simulink model "exampleModel_bus_axi"  (R2017b)
settings: Solver=VariableStepAuto  StartTime=0.0  StopTime=3e-5  RelTol=1e-3
PreLoadFcn:
  | setup
values from neighbouring files (symbols this model uses):
  axiClk = 156.25e6    (= 156250000)    [setup.m]    (also in setup_exampleModel_bus_axi_simulink.m; setup_exampleModel_bus_axi_simulink_lcls2.m; setup_lcls2_pcav.m; sysgen_signal.m)
  cav1p1_addr = 204    [setup_exampleModel_bus_axi_simulink.m]    (also in setup_exampleModel_bus_axi_simulink_lcls2.m; setup_lcls2_pcav.m; sysgen_signal.m)
  cav1p2_addr = cav1p1_addr * 2    (= 408)    [setup_exampleModel_bus_axi_simulink.m]    (also in setup_exampleModel_bus_axi_simulink_lcls2.m; setup_lcls2_pcav.m; sysgen_signal.m)
  cav2p1_addr = cav1p1_addr * 3    (= 612)    [setup_exampleModel_bus_axi_simulink.m]    (also in setup_exampleModel_bus_axi_simulink_lcls2.m; setup_lcls2_pcav.m; sysgen_signal.m)
  cav2p2_addr = cav1p1_addr * 4    (= 816)    [setup_exampleModel_bus_axi_simulink.m]    (also in setup_exampleModel_bus_axi_simulink_lcls2.m; setup_lcls2_pcav.m; sysgen_signal.m)
  Fadc = Fs/interleavedChannels    (= 29750000)    [setup.m]    (also in setup_exampleModel_bus_axi_simulink.m = 357000000; setup_exampleModel_bus_axi_simulink_lcls2.m = 351000000; setup_lcls2_pcav.m = 357000000; sysgen_signal.m = 357000000)
  Fproc = 204e6    (= 204000000)    [setup_exampleModel_bus_axi_simulink.m]    (also in setup_exampleModel_bus_axi_simulink_lcls2.m = 200571400; setup_lcls2_pcav.m; sysgen_signal.m)
  Fsig = Fproc/12    (= 17000000)    [setup_exampleModel_bus_axi_simulink.m]    (also in setup_exampleModel_bus_axi_simulink_lcls2.m = 16714283.3333; setup_lcls2_pcav.m)
  Tadc = 1/fadc    (= 2.80112044818e-09)    [cavity_signal.m]    (also in setup_exampleModel_bus_axi_simulink.m; setup_exampleModel_bus_axi_simulink_lcls2.m = 2.849002849e-09; setup_lcls2_pcav.m; setup_pcav_simulink.m)
undefined symbols (not defined in the file or in its folder): AXI4, Lite
libraries: xbsIndex_r4 x2037, llrf_lib x10, simulink x1
(part 11 of 12)

== system exampleModel_bus_axi/example/dsp/Cav1/c1p2_freq_err_module1/freq_err1/delta_phi ==
  note: calculating delta phi
  phase : Inport
  window : Inport  Port=2
  reset : Inport  Port=3
  AddSub3 : xbsIndex_r4/AddSub  mode=Subtraction  use_carryin=off  use_carryout=off  en=on  latency=1  precision=Full  arith_type="Signed  (2's comp)"  n_bits=32  bin_pt=30  quantization=Truncate  overflow=Saturate  use_behavioral_HDL=off  hw_selection=Fabric  pipelined=off  dbl_ovrd=off  block_type=addsub
  Constant : xbsIndex_r4/Constant  const=0  gui_display_data_type=Fixed-point  arith_type=Signed (2's comp)  n_bits=1  bin_pt=0  preci_type=Single  exp_width=8  frac_width=24  explicit_period=off  period=1  equ=P=C  opselect=C  inp2=PCIN>>17  opr=+  inp1=P  carry=CIN  dbl_ovrd=off  block_type=constant
  Constant1 : xbsIndex_r4/Constant  const=0  gui_display_data_type=Fixed-point  arith_type=Signed (2's comp)  n_bits=1  bin_pt=0  preci_type=Single  exp_width=8  frac_width=24  explicit_period=off  period=1  equ=P=C  opselect=C  inp2=PCIN>>17  opr=+  inp1=P  carry=CIN  dbl_ovrd=off  block_type=constant
  Convert1 : xbsIndex_r4/Convert  gui_display_data_type=Boolean  arith_type=Boolean  n_bits=16  bin_pt=14  float_type=Single  exp_bits=8  fraction_bits=24  quantization=Truncate  overflow=Wrap  en=off  latency=1  pipeline=off  dbl_ovrd=off  block_type=convert
  Delay : xbsIndex_r4/Delay  rst=off  infoeditControl=Selection of Reset will increase slice count due to use of real FFs and instead of SRLs  en=off  latency=5  reg_retiming=off  dbl_ovrd=off  block_type=delay
  Delay2 : xbsIndex_r4/Delay  rst=off  infoeditControl=Selection of Reset will increase slice count due to use of real FFs and instead of SRLs  en=off  latency=2  reg_retiming=off  dbl_ovrd=off  block_type=delay
  Display : Display
  Display1 : Display
  Display2 : Display
  Gateway Out27 : xbsIndex_r4/Gateway Out  inherit_from_input=off  hdl_port=on  rows=1  columns=1  UseAsDAC=off  DACChannel='1'  interface=None  automatic_assignment=on  address_offset=hex2dec('00')  intf_name=''  intf_description=''  timing_constraint=None  locs_specified=off  LOCs={}  io_standard={}  block_type=gatewayout
  Gateway Out28 : xbsIndex_r4/Gateway Out  inherit_from_input=off  hdl_port=on  rows=1  columns=1  UseAsDAC=off  DACChannel='1'  interface=None  automatic_assignment=on  address_offset=hex2dec('00')  intf_name=''  intf_description=''  timing_constraint=None  locs_specified=off  LOCs={}  io_standard={}  block_type=gatewayout
  Gateway Out29 : xbsIndex_r4/Gateway Out  inherit_from_input=off  hdl_port=on  rows=1  columns=1  UseAsDAC=off  DACChannel='1'  interface=None  automatic_assignment=on  address_offset=hex2dec('00')  intf_name=''  intf_description=''  timing_constraint=None  locs_specified=off  LOCs={}  io_standard={}  block_type=gatewayout
  Inverter : xbsIndex_r4/Inverter  en=off  latency=1  dbl_ovrd=off  block_type=inv
  Logical : xbsIndex_r4/Logical  logical_function=AND  inputs=2  en=off  latency=7  precision=User Defined  arith_type=Boolean  n_bits=1  bin_pt=0  align_bp=on  dbl_ovrd=off  block_type=logical
  Relational : xbsIndex_r4/Relational  mode=a!=b  op_type=Bool  en=off  latency=1  dbl_ovrd=off  block_type=relational
  Relational1 : xbsIndex_r4/Relational  mode=a!=b  op_type=Bool  en=off  latency=1  dbl_ovrd=off  block_type=relational
  low_bit : Scope  NumInputPorts=4
  phase_latching : Subsystem
  posedge_pulse : Subsystem
  d_phi : Outport
  val_latched : Outport  Port=2
  wires:
  Delay/1 -> val_latched/1
  posedge_pulse/1(Out1) -> Delay/1
  reset/1 -> phase_latching/3(reset)
  Inverter/1 -> Delay2/1
  Delay2/1 -> AddSub3/3
  Gateway Out29/1 -> low_bit/1, Display/1
  phase/1 -> phase_latching/1(phase)
  AddSub3/1 -> Gateway Out27/1, d_phi/1
  Gateway Out28/1 -> low_bit/2, Display1/1
  Gateway Out27/1 -> low_bit/3, Display2/1
  Convert1/1 -> Inverter/1
  window/1 -> Convert1/1, phase_latching/2(window)
  phase_latching/1(Stop_value) -> AddSub3/1, Relational/1, Gateway Out29/1
  Constant/1 -> Relational/2
  Constant1/1 -> Relational1/2
  phase_latching/2(Start_value) -> Relational1/1, Gateway Out28/1, AddSub3/2
  Relational/1 -> Logical/1
  Relational1/1 -> Logical/2
  Logical/1 -> posedge_pulse/1(In1)

== system exampleModel_bus_axi/example/dsp/Cav1/c1p2_freq_err_module1/freq_err1/delta_t ==
  note: (2*pi)/(17E6)
  window : Inport
  reset : Inport  Port=2
  Constant1 : xbsIndex_r4/Constant  const=2*pi*(1/(Fsig))  gui_display_data_type=Fixed-point  arith_type=Unsigned  n_bits=42  bin_pt=42  preci_type=Single  exp_width=8  frac_width=24  explicit_period=off  period=1  equ=P=C  opselect=C  inp2=PCIN>>17  opr=+  inp1=P  carry=CIN  dbl_ovrd=off  block_type=constant
  Convert1 : xbsIndex_r4/Convert  gui_display_data_type=Boolean  arith_type=Boolean  n_bits=16  bin_pt=14  float_type=Single  exp_bits=8  fraction_bits=24  quantization=Truncate  overflow=Wrap  en=off  latency=1  pipeline=off  dbl_ovrd=off  block_type=convert
  Counter2 : xbsIndex_r4/Counter  cnt_type=Free Running  cnt_to=Inf  operation=Up  start_count=1  cnt_by_val=1  arith_type=Unsigned  n_bits=10  bin_pt=0  load_pin=off  rst=on  en=on  explicit_period=on  period=1/(17e6)  use_behavioral_HDL=off  implementation=Fabric  dbl_ovrd=off  block_type=counter
  Delay : xbsIndex_r4/Delay  rst=off  infoeditControl=Selection of Reset will increase slice count due to use of real FFs and instead of SRLs  en=off  latency=1  reg_retiming=off  dbl_ovrd=off  block_type=delay
  Display1 : Display
  Display3 : Display
  Gateway Out1 : xbsIndex_r4/Gateway Out  inherit_from_input=off  hdl_port=on  rows=1  columns=1  UseAsDAC=off  DACChannel='1'  interface=None  automatic_assignment=on  address_offset=hex2dec('00')  intf_name=''  intf_description=''  timing_constraint=None  locs_specified=off  LOCs={}  io_standard={}  block_type=gatewayout
  Gateway Out6 : xbsIndex_r4/Gateway Out  inherit_from_input=off  hdl_port=on  rows=1  columns=1  UseAsDAC=off  DACChannel='1'  interface=None  automatic_assignment=on  address_offset=hex2dec('00')  intf_name=''  intf_description=''  timing_constraint=None  locs_specified=off  LOCs={}  io_standard={}  block_type=gatewayout
  Mult1 : xbsIndex_r4/Mult  precision=User Defined  arith_type="Signed  (2's comp)"  n_bits=32  bin_pt=32  quantization=Truncate  overflow=Saturate  en=off  latency=3  use_behavioral_HDL=off  opt=Speed  use_embedded=on  optimum_pipeline=off  pipeline=on  dbl_ovrd=off  use_rpm=on  placement_style=Triangular  block_type=mult
  Register2 : xbsIndex_r4/Register  init=0  rst=on  en=on  dbl_ovrd=off  block_type=register
  dt : Outport
  wires:
  Constant1/1 -> Mult1/2
  Mult1/1 -> dt/1, Gateway Out1/1
  reset/1 -> Register2/2, Counter2/1
  Register2/1 -> Gateway Out6/1, Mult1/1
  Counter2/1 -> Register2/1
  window/1 -> Convert1/1
  Gateway Out1/1 -> Display3/1
  Gateway Out6/1 -> Display1/1
  Convert1/1 -> Delay/1
  Delay/1 -> Register2/3, Counter2/2

== system exampleModel_bus_axi/example/dsp/Cav1/c1p2_freq_err_module1/freq_err1/negedge_pulse ==
  In1 : Inport
  Delay3 : xbsIndex_r4/Delay  rst=off  infoeditControl=Selection of Reset will increase slice count due to use of real FFs and instead of SRLs  en=off  latency=4  reg_retiming=off  dbl_ovrd=off  block_type=delay
  Inverter : xbsIndex_r4/Inverter  en=off  latency=1  dbl_ovrd=off  block_type=inv
  Logical : xbsIndex_r4/Logical  logical_function=AND  inputs=2  en=off  latency=1  precision=Full  arith_type=Unsigned  n_bits=16  bin_pt=0  align_bp=on  dbl_ovrd=off  block_type=logical
  Out1 : Outport
  wires:
  Delay3/1 -> Logical/2
  Logical/1 -> Out1/1
  Inverter/1 -> Logical/1
  In1/1 -> Delay3/1, Inverter/1

== system exampleModel_bus_axi/example/dsp/Cav1/c1p2_freq_err_module1/freq_err1/posedge_pulse ==
  In1 : Inport
  Inverter1 : xbsIndex_r4/Inverter  en=off  latency=1  dbl_ovrd=off  block_type=inv
  Logical : xbsIndex_r4/Logical  logical_function=AND  inputs=2  en=off  latency=1  precision=Full  arith_type=Unsigned  n_bits=16  bin_pt=0  align_bp=on  dbl_ovrd=off  block_type=logical
  Out1 : Outport
  wires:
  In1/1 -> Logical/1, Inverter1/1
  Logical/1 -> Out1/1
  Inverter1/1 -> Logical/2

== system exampleModel_bus_axi/example/dsp/Cav1/c1p2_freq_err_module2/freq_err1/delta_phi ==
  note: calculating delta phi
  phase : Inport
  window : Inport  Port=2
  reset : Inport  Port=3
  AddSub3 : xbsIndex_r4/AddSub  mode=Subtraction  use_carryin=off  use_carryout=off  en=on  latency=1  precision=Full  arith_type="Signed  (2's comp)"  n_bits=32  bin_pt=30  quantization=Truncate  overflow=Saturate  use_behavioral_HDL=off  hw_selection=Fabric  pipelined=off  dbl_ovrd=off  block_type=addsub
  Constant : xbsIndex_r4/Constant  const=0  gui_display_data_type=Fixed-point  arith_type=Signed (2's comp)  n_bits=1  bin_pt=0  preci_type=Single  exp_width=8  frac_width=24  explicit_period=off  period=1  equ=P=C  opselect=C  inp2=PCIN>>17  opr=+  inp1=P  carry=CIN  dbl_ovrd=off  block_type=constant
  Constant1 : xbsIndex_r4/Constant  const=0  gui_display_data_type=Fixed-point  arith_type=Signed (2's comp)  n_bits=1  bin_pt=0  preci_type=Single  exp_width=8  frac_width=24  explicit_period=off  period=1  equ=P=C  opselect=C  inp2=PCIN>>17  opr=+  inp1=P  carry=CIN  dbl_ovrd=off  block_type=constant
  Convert1 : xbsIndex_r4/Convert  gui_display_data_type=Boolean  arith_type=Boolean  n_bits=16  bin_pt=14  float_type=Single  exp_bits=8  fraction_bits=24  quantization=Truncate  overflow=Wrap  en=off  latency=1  pipeline=off  dbl_ovrd=off  block_type=convert
  Delay : xbsIndex_r4/Delay  rst=off  infoeditControl=Selection of Reset will increase slice count due to use of real FFs and instead of SRLs  en=off  latency=5  reg_retiming=off  dbl_ovrd=off  block_type=delay
  Delay2 : xbsIndex_r4/Delay  rst=off  infoeditControl=Selection of Reset will increase slice count due to use of real FFs and instead of SRLs  en=off  latency=2  reg_retiming=off  dbl_ovrd=off  block_type=delay
  Display : Display
  Display1 : Display
  Display2 : Display
  Gateway Out27 : xbsIndex_r4/Gateway Out  inherit_from_input=off  hdl_port=on  rows=1  columns=1  UseAsDAC=off  DACChannel='1'  interface=None  automatic_assignment=on  address_offset=hex2dec('00')  intf_name=''  intf_description=''  timing_constraint=None  locs_specified=off  LOCs={}  io_standard={}  block_type=gatewayout
  Gateway Out28 : xbsIndex_r4/Gateway Out  inherit_from_input=off  hdl_port=on  rows=1  columns=1  UseAsDAC=off  DACChannel='1'  interface=None  automatic_assignment=on  address_offset=hex2dec('00')  intf_name=''  intf_description=''  timing_constraint=None  locs_specified=off  LOCs={}  io_standard={}  block_type=gatewayout
  Gateway Out29 : xbsIndex_r4/Gateway Out  inherit_from_input=off  hdl_port=on  rows=1  columns=1  UseAsDAC=off  DACChannel='1'  interface=None  automatic_assignment=on  address_offset=hex2dec('00')  intf_name=''  intf_description=''  timing_constraint=None  locs_specified=off  LOCs={}  io_standard={}  block_type=gatewayout
  Inverter : xbsIndex_r4/Inverter  en=off  latency=1  dbl_ovrd=off  block_type=inv
  Logical : xbsIndex_r4/Logical  logical_function=AND  inputs=2  en=off  latency=7  precision=User Defined  arith_type=Boolean  n_bits=1  bin_pt=0  align_bp=on  dbl_ovrd=off  block_type=logical
  Relational : xbsIndex_r4/Relational  mode=a!=b  op_type=Bool  en=off  latency=1  dbl_ovrd=off  block_type=relational
  Relational1 : xbsIndex_r4/Relational  mode=a!=b  op_type=Bool  en=off  latency=1  dbl_ovrd=off  block_type=relational
  low_bit : Scope  NumInputPorts=4
  phase_latching : Subsystem
  posedge_pulse : Subsystem
  d_phi : Outport
  val_latched : Outport  Port=2
  wires:
  Delay/1 -> val_latched/1
  posedge_pulse/1(Out1) -> Delay/1
  reset/1 -> phase_latching/3(reset)
  Inverter/1 -> Delay2/1
  Delay2/1 -> AddSub3/3
  Gateway Out29/1 -> low_bit/1, Display/1
  phase/1 -> phase_latching/1(phase)
  AddSub3/1 -> Gateway Out27/1, d_phi/1
  Gateway Out28/1 -> low_bit/2, Display1/1
  Gateway Out27/1 -> low_bit/3, Display2/1
  Convert1/1 -> Inverter/1
  window/1 -> Convert1/1, phase_latching/2(window)
  phase_latching/1(Stop_value) -> AddSub3/1, Relational/1, Gateway Out29/1
  Constant/1 -> Relational/2
  Constant1/1 -> Relational1/2
  phase_latching/2(Start_value) -> Relational1/1, Gateway Out28/1, AddSub3/2
  Relational/1 -> Logical/1
  Relational1/1 -> Logical/2
  Logical/1 -> posedge_pulse/1(In1)

== system exampleModel_bus_axi/example/dsp/Cav1/c1p2_freq_err_module2/freq_err1/delta_t ==
  note: (2*pi)/(17E6)
  window : Inport
  reset : Inport  Port=2
  Constant1 : xbsIndex_r4/Constant  const=2*pi*(1/(Fsig))  gui_display_data_type=Fixed-point  arith_type=Unsigned  n_bits=42  bin_pt=42  preci_type=Single  exp_width=8  frac_width=24  explicit_period=off  period=1  equ=P=C  opselect=C  inp2=PCIN>>17  opr=+  inp1=P  carry=CIN  dbl_ovrd=off  block_type=constant
  Convert1 : xbsIndex_r4/Convert  gui_display_data_type=Boolean  arith_type=Boolean  n_bits=16  bin_pt=14  float_type=Single  exp_bits=8  fraction_bits=24  quantization=Truncate  overflow=Wrap  en=off  latency=1  pipeline=off  dbl_ovrd=off  block_type=convert
  Counter2 : xbsIndex_r4/Counter  cnt_type=Free Running  cnt_to=Inf  operation=Up  start_count=1  cnt_by_val=1  arith_type=Unsigned  n_bits=10  bin_pt=0  load_pin=off  rst=on  en=on  explicit_period=on  period=1/(17e6)  use_behavioral_HDL=off  implementation=Fabric  dbl_ovrd=off  block_type=counter
  Delay : xbsIndex_r4/Delay  rst=off  infoeditControl=Selection of Reset will increase slice count due to use of real FFs and instead of SRLs  en=off  latency=1  reg_retiming=off  dbl_ovrd=off  block_type=delay
  Display1 : Display
  Display3 : Display
  Gateway Out1 : xbsIndex_r4/Gateway Out  inherit_from_input=off  hdl_port=on  rows=1  columns=1  UseAsDAC=off  DACChannel='1'  interface=None  automatic_assignment=on  address_offset=hex2dec('00')  intf_name=''  intf_description=''  timing_constraint=None  locs_specified=off  LOCs={}  io_standard={}  block_type=gatewayout
  Gateway Out6 : xbsIndex_r4/Gateway Out  inherit_from_input=off  hdl_port=on  rows=1  columns=1  UseAsDAC=off  DACChannel='1'  interface=None  automatic_assignment=on  address_offset=hex2dec('00')  intf_name=''  intf_description=''  timing_constraint=None  locs_specified=off  LOCs={}  io_standard={}  block_type=gatewayout
  Mult1 : xbsIndex_r4/Mult  precision=User Defined  arith_type="Signed  (2's comp)"  n_bits=32  bin_pt=32  quantization=Truncate  overflow=Saturate  en=off  latency=3  use_behavioral_HDL=off  opt=Speed  use_embedded=on  optimum_pipeline=off  pipeline=on  dbl_ovrd=off  use_rpm=on  placement_style=Triangular  block_type=mult
  Register2 : xbsIndex_r4/Register  init=0  rst=on  en=on  dbl_ovrd=off  block_type=register
  dt : Outport
  wires:
  Constant1/1 -> Mult1/2
  Mult1/1 -> dt/1, Gateway Out1/1
  reset/1 -> Register2/2, Counter2/1
  Register2/1 -> Gateway Out6/1, Mult1/1
  Counter2/1 -> Register2/1
  window/1 -> Convert1/1
  Gateway Out1/1 -> Display3/1
  Gateway Out6/1 -> Display1/1
  Convert1/1 -> Delay/1
  Delay/1 -> Register2/3, Counter2/2

== system exampleModel_bus_axi/example/dsp/Cav1/c1p2_freq_err_module2/freq_err1/negedge_pulse ==
  In1 : Inport
  Delay3 : xbsIndex_r4/Delay  rst=off  infoeditControl=Selection of Reset will increase slice count due to use of real FFs and instead of SRLs  en=off  latency=4  reg_retiming=off  dbl_ovrd=off  block_type=delay
  Inverter : xbsIndex_r4/Inverter  en=off  latency=1  dbl_ovrd=off  block_type=inv
  Logical : xbsIndex_r4/Logical  logical_function=AND  inputs=2  en=off  latency=1  precision=Full  arith_type=Unsigned  n_bits=16  bin_pt=0  align_bp=on  dbl_ovrd=off  block_type=logical
  Out1 : Outport
  wires:
  Delay3/1 -> Logical/2
  Logical/1 -> Out1/1
  Inverter/1 -> Logical/1
  In1/1 -> Delay3/1, Inverter/1

== system exampleModel_bus_axi/example/dsp/Cav1/c1p2_freq_err_module2/freq_err1/posedge_pulse ==
  In1 : Inport
  Inverter1 : xbsIndex_r4/Inverter  en=off  latency=1  dbl_ovrd=off  block_type=inv
  Logical : xbsIndex_r4/Logical  logical_function=AND  inputs=2  en=off  latency=1  precision=Full  arith_type=Unsigned  n_bits=16  bin_pt=0  align_bp=on  dbl_ovrd=off  block_type=logical
  Out1 : Outport
  wires:
  In1/1 -> Logical/1, Inverter1/1
  Logical/1 -> Out1/1
  Inverter1/1 -> Logical/2

== system exampleModel_bus_axi/example/dsp/Cav2/IQ_integration1/IQ_latch_normalize/Subsystem ==
  I : Inport
  Q : Inport  Port=2
  Absolute : xbsIndex_r4/Absolute  precision=Full  arith_type=Unsigned  n_bits=16  bin_pt=14  quantization=Truncate  overflow=Wrap  en=off  latency=1  dbl_ovrd=off  block_type=abs
  Absolute1 : xbsIndex_r4/Absolute  precision=Full  arith_type=Unsigned  n_bits=16  bin_pt=14  quantization=Truncate  overflow=Wrap  en=off  latency=1  dbl_ovrd=off  block_type=abs
  Convert4 : xbsIndex_r4/Convert  gui_display_data_type=Fixed-point  arith_type="Signed  (2's comp)"  n_bits=18  bin_pt=16  float_type=Single  exp_bits=8  fraction_bits=24  quantization=Truncate  overflow=Wrap  en=off  latency=1  pipeline=off  dbl_ovrd=off  block_type=convert
  Convert9 : xbsIndex_r4/Convert  gui_display_data_type=Fixed-point  arith_type="Signed  (2's comp)"  n_bits=18  bin_pt=16  float_type=Single  exp_bits=8  fraction_bits=24  quantization=Truncate  overflow=Wrap  en=off  latency=1  pipeline=off  dbl_ovrd=off  block_type=convert
  Delay : xbsIndex_r4/Delay  rst=off  infoeditControl=Selection of Reset will increase slice count due to use of real FFs and instead of SRLs  en=off  latency=1  reg_retiming=off  dbl_ovrd=off  block_type=delay
  Delay1 : xbsIndex_r4/Delay  rst=off  infoeditControl=Selection of Reset will increase slice count due to use of real FFs and instead of SRLs  en=off  latency=1  reg_retiming=off  dbl_ovrd=off  block_type=delay
  Display2 : Display
  Gateway Out{1..6,22,24,27} (9 alike) : xbsIndex_r4/Gateway Out  inherit_from_input=off  hdl_port=on  rows=1  columns=1  UseAsDAC=off  DACChannel='1'  interface=None  automatic_assignment=on  address_offset=hex2dec('00')  intf_name=''  intf_description=''  timing_constraint=None  locs_specified=off  LOCs={}  io_standard={}  block_type=gatewayout
  MCode : xbsIndex_r4/MCode  mfname=integration_normalize  explicit_period=off  period=1  inputsTable={'boundInpExpr'=>['','','',''],'inputs'=>['I_int','Q_int','I_int_abs','Q_int_abs']}  outputsTable={'outputs'=>['I_norm','Q_norm','done','bit'],'suppressOut'=>['off','off','off','off']}  enable_stdout=off  enable_debug=off  suppress_output=on  defparams={}  hide_port_list={}  dbl_ovrd=off  block_type=mcode
  Scope1 : Scope  NumInputPorts=4
  Scope11 : Scope  NumInputPorts=4
  I_norm : Outport
  Q_norm : Outport  Port=2
  done : Outport  Port=3
  bit : Outport  Port=4
  wires:
  MCode/3 -> done/1
  Absolute1/1 -> MCode/4
  Gateway Out22/1 -> Scope11/2
  Delay1/1 -> Gateway Out6/1, MCode/2
  Q/1 -> Delay1/1, Absolute1/1
  Absolute/1 -> MCode/3
  MCode/4 -> bit/1, Gateway Out27/1
  I/1 -> Absolute/1, Delay/1
  MCode/2 -> Gateway Out5/1, Gateway Out4/1, Convert4/1
  Gateway Out24/1 -> Scope11/1
  Gateway Out27/1 -> Display2/1
  Delay/1 -> Gateway Out24/1, MCode/1
  MCode/1 -> Gateway Out3/1, Convert9/1, Gateway Out22/1
  Convert4/1 -> Q_norm/1, Gateway Out1/1
  Convert9/1 -> I_norm/1, Gateway Out2/1
  Gateway Out1/1 -> Scope1/2
  Gateway Out2/1 -> Scope1/4
  Gateway Out4/1 -> Scope1/1
  Gateway Out3/1 -> Scope1/3
  Gateway Out6/1 -> Scope11/3
  Gateway Out5/1 -> Scope11/4

== system exampleModel_bus_axi/example/dsp/Cav2/IQ_integration1/IQ_latch_normalize/Subsystem4 ==
  d : Inport
  reset : Inport  Port=2
  Latch : Inport  Port=3
  Register11 : xbsIndex_r4/Register  init=0  rst=on  en=on  dbl_ovrd=off  block_type=register
  posedge_pulse : Subsystem
  q : Outport
  wires:
  d/1 -> Register11/1
  Register11/1 -> q/1
  posedge_pulse/1(Out1) -> Register11/3
  Latch/1 -> posedge_pulse/1(In1)
  reset/1 -> Register11/2

== system exampleModel_bus_axi/example/dsp/Cav2/IQ_integration1/IQ_latch_normalize/Subsystem5 ==
  d : Inport
  reset : Inport  Port=2
  Latch : Inport  Port=3
  Register11 : xbsIndex_r4/Register  init=0  rst=on  en=on  dbl_ovrd=off  block_type=register
  posedge_pulse : Subsystem
  q : Outport
  wires:
  reset/1 -> Register11/2
  Latch/1 -> posedge_pulse/1(In1)
  posedge_pulse/1(Out1) -> Register11/3
  Register11/1 -> q/1
  d/1 -> Register11/1

== system exampleModel_bus_axi/example/dsp/Cav2/IQ_integration1/IQ_latch_normalize1/Subsystem ==
  I : Inport
  Q : Inport  Port=2
  Absolute : xbsIndex_r4/Absolute  precision=Full  arith_type=Unsigned  n_bits=16  bin_pt=14  quantization=Truncate  overflow=Wrap  en=off  latency=1  dbl_ovrd=off  block_type=abs
  Absolute1 : xbsIndex_r4/Absolute  precision=Full  arith_type=Unsigned  n_bits=16  bin_pt=14  quantization=Truncate  overflow=Wrap  en=off  latency=1  dbl_ovrd=off  block_type=abs
  Convert4 : xbsIndex_r4/Convert  gui_display_data_type=Fixed-point  arith_type="Signed  (2's comp)"  n_bits=18  bin_pt=16  float_type=Single  exp_bits=8  fraction_bits=24  quantization=Truncate  overflow=Wrap  en=off  latency=1  pipeline=off  dbl_ovrd=off  block_type=convert
  Convert9 : xbsIndex_r4/Convert  gui_display_data_type=Fixed-point  arith_type="Signed  (2's comp)"  n_bits=18  bin_pt=16  float_type=Single  exp_bits=8  fraction_bits=24  quantization=Truncate  overflow=Wrap  en=off  latency=1  pipeline=off  dbl_ovrd=off  block_type=convert
  Delay : xbsIndex_r4/Delay  rst=off  infoeditControl=Selection of Reset will increase slice count due to use of real FFs and instead of SRLs  en=off  latency=1  reg_retiming=off  dbl_ovrd=off  block_type=delay
  Delay1 : xbsIndex_r4/Delay  rst=off  infoeditControl=Selection of Reset will increase slice count due to use of real FFs and instead of SRLs  en=off  latency=1  reg_retiming=off  dbl_ovrd=off  block_type=delay
  Display2 : Display
  Gateway Out{1..6,22,24,27} (9 alike) : xbsIndex_r4/Gateway Out  inherit_from_input=off  hdl_port=on  rows=1  columns=1  UseAsDAC=off  DACChannel='1'  interface=None  automatic_assignment=on  address_offset=hex2dec('00')  intf_name=''  intf_description=''  timing_constraint=None  locs_specified=off  LOCs={}  io_standard={}  block_type=gatewayout
  MCode : xbsIndex_r4/MCode  mfname=integration_normalize  explicit_period=off  period=1  inputsTable={'boundInpExpr'=>['','','',''],'inputs'=>['I_int','Q_int','I_int_abs','Q_int_abs']}  outputsTable={'outputs'=>['I_norm','Q_norm','done','bit'],'suppressOut'=>['off','off','off','off']}  enable_stdout=off  enable_debug=off  suppress_output=on  defparams={}  hide_port_list={}  dbl_ovrd=off  block_type=mcode
  Scope1 : Scope  NumInputPorts=4
  Scope11 : Scope  NumInputPorts=4
  I_norm : Outport
  Q_norm : Outport  Port=2
  done : Outport  Port=3
  bit : Outport  Port=4
  wires:
  Gateway Out5/1 -> Scope11/4
  Gateway Out6/1 -> Scope11/3
  Gateway Out3/1 -> Scope1/3
  Gateway Out4/1 -> Scope1/1
  Gateway Out2/1 -> Scope1/4
  Gateway Out1/1 -> Scope1/2
  Convert9/1 -> Gateway Out2/1, I_norm/1
  Convert4/1 -> Gateway Out1/1, Q_norm/1
  MCode/1 -> Gateway Out22/1, Convert9/1, Gateway Out3/1
  Delay/1 -> MCode/1, Gateway Out24/1
  Gateway Out27/1 -> Display2/1
  Gateway Out24/1 -> Scope11/1
  MCode/2 -> Convert4/1, Gateway Out4/1, Gateway Out5/1
  I/1 -> Delay/1, Absolute/1
  MCode/4 -> Gateway Out27/1, bit/1
  Absolute/1 -> MCode/3
  Q/1 -> Absolute1/1, Delay1/1
  Delay1/1 -> MCode/2, Gateway Out6/1
  Gateway Out22/1 -> Scope11/2
  Absolute1/1 -> MCode/4
  MCode/3 -> done/1

== system exampleModel_bus_axi/example/dsp/Cav2/IQ_integration1/IQ_latch_normalize1/Subsystem4 ==
  d : Inport
  reset : Inport  Port=2
  Latch : Inport  Port=3
  Register11 : xbsIndex_r4/Register  init=0  rst=on  en=on  dbl_ovrd=off  block_type=register
  posedge_pulse : Subsystem
  q : Outport
  wires:
  reset/1 -> Register11/2
  Latch/1 -> posedge_pulse/1(In1)
  posedge_pulse/1(Out1) -> Register11/3
  Register11/1 -> q/1
  d/1 -> Register11/1

== system exampleModel_bus_axi/example/dsp/Cav2/IQ_integration1/IQ_latch_normalize1/Subsystem5 ==
  d : Inport
  reset : Inport  Port=2
  Latch : Inport  Port=3
  Register11 : xbsIndex_r4/Register  init=0  rst=on  en=on  dbl_ovrd=off  block_type=register
  posedge_pulse : Subsystem
  q : Outport
  wires:
  d/1 -> Register11/1
  Register11/1 -> q/1
  posedge_pulse/1(Out1) -> Register11/3
  Latch/1 -> posedge_pulse/1(In1)
  reset/1 -> Register11/2

== system exampleModel_bus_axi/example/dsp/Cav2/IQ_integration2/IQ_latch_normalize/Subsystem ==
  I : Inport
  Q : Inport  Port=2
  Absolute : xbsIndex_r4/Absolute  precision=Full  arith_type=Unsigned  n_bits=16  bin_pt=14  quantization=Truncate  overflow=Wrap  en=off  latency=1  dbl_ovrd=off  block_type=abs
  Absolute1 : xbsIndex_r4/Absolute  precision=Full  arith_type=Unsigned  n_bits=16  bin_pt=14  quantization=Truncate  overflow=Wrap  en=off  latency=1  dbl_ovrd=off  block_type=abs
  Convert4 : xbsIndex_r4/Convert  gui_display_data_type=Fixed-point  arith_type="Signed  (2's comp)"  n_bits=18  bin_pt=16  float_type=Single  exp_bits=8  fraction_bits=24  quantization=Truncate  overflow=Wrap  en=off  latency=1  pipeline=off  dbl_ovrd=off  block_type=convert
  Convert9 : xbsIndex_r4/Convert  gui_display_data_type=Fixed-point  arith_type="Signed  (2's comp)"  n_bits=18  bin_pt=16  float_type=Single  exp_bits=8  fraction_bits=24  quantization=Truncate  overflow=Wrap  en=off  latency=1  pipeline=off  dbl_ovrd=off  block_type=convert
  Delay : xbsIndex_r4/Delay  rst=off  infoeditControl=Selection of Reset will increase slice count due to use of real FFs and instead of SRLs  en=off  latency=1  reg_retiming=off  dbl_ovrd=off  block_type=delay
  Delay1 : xbsIndex_r4/Delay  rst=off  infoeditControl=Selection of Reset will increase slice count due to use of real FFs and instead of SRLs  en=off  latency=1  reg_retiming=off  dbl_ovrd=off  block_type=delay
  Display2 : Display
  Gateway Out{1..6,22,24,27} (9 alike) : xbsIndex_r4/Gateway Out  inherit_from_input=off  hdl_port=on  rows=1  columns=1  UseAsDAC=off  DACChannel='1'  interface=None  automatic_assignment=on  address_offset=hex2dec('00')  intf_name=''  intf_description=''  timing_constraint=None  locs_specified=off  LOCs={}  io_standard={}  block_type=gatewayout
  MCode : xbsIndex_r4/MCode  mfname=integration_normalize  explicit_period=off  period=1  inputsTable={'boundInpExpr'=>['','','',''],'inputs'=>['I_int','Q_int','I_int_abs','Q_int_abs']}  outputsTable={'outputs'=>['I_norm','Q_norm','done','bit'],'suppressOut'=>['off','off','off','off']}  enable_stdout=off  enable_debug=off  suppress_output=on  defparams={}  hide_port_list={}  dbl_ovrd=off  block_type=mcode
  Scope1 : Scope  NumInputPorts=4
  Scope11 : Scope  NumInputPorts=4
  I_norm : Outport
  Q_norm : Outport  Port=2
  done : Outport  Port=3
  bit : Outport  Port=4
  wires:
  MCode/3 -> done/1
  Absolute1/1 -> MCode/4
  Gateway Out22/1 -> Scope11/2
  Delay1/1 -> Gateway Out6/1, MCode/2
  Q/1 -> Delay1/1, Absolute1/1
  Absolute/1 -> MCode/3
  MCode/4 -> bit/1, Gateway Out27/1
  I/1 -> Absolute/1, Delay/1
  MCode/2 -> Gateway Out5/1, Gateway Out4/1, Convert4/1
  Gateway Out24/1 -> Scope11/1
  Gateway Out27/1 -> Display2/1
  Delay/1 -> Gateway Out24/1, MCode/1
  MCode/1 -> Gateway Out3/1, Convert9/1, Gateway Out22/1
  Convert4/1 -> Q_norm/1, Gateway Out1/1
  Convert9/1 -> I_norm/1, Gateway Out2/1
  Gateway Out1/1 -> Scope1/2
  Gateway Out2/1 -> Scope1/4
  Gateway Out4/1 -> Scope1/1
  Gateway Out3/1 -> Scope1/3
  Gateway Out6/1 -> Scope11/3
  Gateway Out5/1 -> Scope11/4

== system exampleModel_bus_axi/example/dsp/Cav2/IQ_integration2/IQ_latch_normalize/Subsystem4 ==
  d : Inport
  reset : Inport  Port=2
  Latch : Inport  Port=3
  Register11 : xbsIndex_r4/Register  init=0  rst=on  en=on  dbl_ovrd=off  block_type=register
  posedge_pulse : Subsystem
  q : Outport
  wires:
  d/1 -> Register11/1
  Register11/1 -> q/1
  posedge_pulse/1(Out1) -> Register11/3
  Latch/1 -> posedge_pulse/1(In1)
  reset/1 -> Register11/2

== system exampleModel_bus_axi/example/dsp/Cav2/IQ_integration2/IQ_latch_normalize/Subsystem5 ==
  d : Inport
  reset : Inport  Port=2
  Latch : Inport  Port=3
  Register11 : xbsIndex_r4/Register  init=0  rst=on  en=on  dbl_ovrd=off  block_type=register
  posedge_pulse : Subsystem
  q : Outport
  wires:
  reset/1 -> Register11/2
  Latch/1 -> posedge_pulse/1(In1)
  posedge_pulse/1(Out1) -> Register11/3
  Register11/1 -> q/1
  d/1 -> Register11/1

== system exampleModel_bus_axi/example/dsp/Cav2/IQ_integration2/IQ_latch_normalize1/Subsystem ==
  I : Inport
  Q : Inport  Port=2
  Absolute : xbsIndex_r4/Absolute  precision=Full  arith_type=Unsigned  n_bits=16  bin_pt=14  quantization=Truncate  overflow=Wrap  en=off  latency=1  dbl_ovrd=off  block_type=abs
  Absolute1 : xbsIndex_r4/Absolute  precision=Full  arith_type=Unsigned  n_bits=16  bin_pt=14  quantization=Truncate  overflow=Wrap  en=off  latency=1  dbl_ovrd=off  block_type=abs
  Convert4 : xbsIndex_r4/Convert  gui_display_data_type=Fixed-point  arith_type="Signed  (2's comp)"  n_bits=18  bin_pt=16  float_type=Single  exp_bits=8  fraction_bits=24  quantization=Truncate  overflow=Wrap  en=off  latency=1  pipeline=off  dbl_ovrd=off  block_type=convert
  Convert9 : xbsIndex_r4/Convert  gui_display_data_type=Fixed-point  arith_type="Signed  (2's comp)"  n_bits=18  bin_pt=16  float_type=Single  exp_bits=8  fraction_bits=24  quantization=Truncate  overflow=Wrap  en=off  latency=1  pipeline=off  dbl_ovrd=off  block_type=convert
  Delay : xbsIndex_r4/Delay  rst=off  infoeditControl=Selection of Reset will increase slice count due to use of real FFs and instead of SRLs  en=off  latency=1  reg_retiming=off  dbl_ovrd=off  block_type=delay
  Delay1 : xbsIndex_r4/Delay  rst=off  infoeditControl=Selection of Reset will increase slice count due to use of real FFs and instead of SRLs  en=off  latency=1  reg_retiming=off  dbl_ovrd=off  block_type=delay
  Display2 : Display
  Gateway Out{1..6,22,24,27} (9 alike) : xbsIndex_r4/Gateway Out  inherit_from_input=off  hdl_port=on  rows=1  columns=1  UseAsDAC=off  DACChannel='1'  interface=None  automatic_assignment=on  address_offset=hex2dec('00')  intf_name=''  intf_description=''  timing_constraint=None  locs_specified=off  LOCs={}  io_standard={}  block_type=gatewayout
  MCode : xbsIndex_r4/MCode  mfname=integration_normalize  explicit_period=off  period=1  inputsTable={'boundInpExpr'=>['','','',''],'inputs'=>['I_int','Q_int','I_int_abs','Q_int_abs']}  outputsTable={'outputs'=>['I_norm','Q_norm','done','bit'],'suppressOut'=>['off','off','off','off']}  enable_stdout=off  enable_debug=off  suppress_output=on  defparams={}  hide_port_list={}  dbl_ovrd=off  block_type=mcode
  Scope1 : Scope  NumInputPorts=4
  Scope11 : Scope  NumInputPorts=4
  I_norm : Outport
  Q_norm : Outport  Port=2
  done : Outport  Port=3
  bit : Outport  Port=4
  wires:
  Gateway Out5/1 -> Scope11/4
  Gateway Out6/1 -> Scope11/3
  Gateway Out3/1 -> Scope1/3
  Gateway Out4/1 -> Scope1/1
  Gateway Out2/1 -> Scope1/4
  Gateway Out1/1 -> Scope1/2
  Convert9/1 -> Gateway Out2/1, I_norm/1
  Convert4/1 -> Gateway Out1/1, Q_norm/1
  MCode/1 -> Gateway Out22/1, Convert9/1, Gateway Out3/1
  Delay/1 -> MCode/1, Gateway Out24/1
  Gateway Out27/1 -> Display2/1
  Gateway Out24/1 -> Scope11/1
  MCode/2 -> Convert4/1, Gateway Out4/1, Gateway Out5/1
  I/1 -> Delay/1, Absolute/1
  MCode/4 -> Gateway Out27/1, bit/1
  Absolute/1 -> MCode/3
  Q/1 -> Absolute1/1, Delay1/1
  Delay1/1 -> MCode/2, Gateway Out6/1
  Gateway Out22/1 -> Scope11/2
  Absolute1/1 -> MCode/4
  MCode/3 -> done/1

== system exampleModel_bus_axi/example/dsp/Cav2/IQ_integration2/IQ_latch_normalize1/Subsystem4 ==
  d : Inport
  reset : Inport  Port=2
  Latch : Inport  Port=3
  Register11 : xbsIndex_r4/Register  init=0  rst=on  en=on  dbl_ovrd=off  block_type=register
  posedge_pulse : Subsystem
  q : Outport
  wires:
  reset/1 -> Register11/2
  Latch/1 -> posedge_pulse/1(In1)
  posedge_pulse/1(Out1) -> Register11/3
  Register11/1 -> q/1
  d/1 -> Register11/1

== system exampleModel_bus_axi/example/dsp/Cav2/IQ_integration2/IQ_latch_normalize1/Subsystem5 ==
  d : Inport
  reset : Inport  Port=2
  Latch : Inport  Port=3
  Register11 : xbsIndex_r4/Register  init=0  rst=on  en=on  dbl_ovrd=off  block_type=register
  posedge_pulse : Subsystem
  q : Outport
  wires:
  d/1 -> Register11/1
  Register11/1 -> q/1
  posedge_pulse/1(Out1) -> Register11/3
  Latch/1 -> posedge_pulse/1(In1)
  reset/1 -> Register11/2

== system exampleModel_bus_axi/example/dsp/Cav2/c1p1_PA_conversion/Subsystem1/posedge_pulse ==
  In1 : Inport
  Inverter1 : xbsIndex_r4/Inverter  en=off  latency=1  dbl_ovrd=off  block_type=inv
  Logical : xbsIndex_r4/Logical  logical_function=AND  inputs=2  en=off  latency=1  precision=Full  arith_type=Unsigned  n_bits=16  bin_pt=0  align_bp=on  dbl_ovrd=off  block_type=logical
  Out1 : Outport
  wires:
  In1/1 -> Logical/1, Inverter1/1
  Logical/1 -> Out1/1
  Inverter1/1 -> Logical/2

== system exampleModel_bus_axi/example/dsp/Cav2/c1p1_PA_conversion/Subsystem2/posedge_pulse ==
  In1 : Inport
  Inverter1 : xbsIndex_r4/Inverter  en=off  latency=1  dbl_ovrd=off  block_type=inv
  Logical : xbsIndex_r4/Logical  logical_function=AND  inputs=2  en=off  latency=1  precision=Full  arith_type=Unsigned  n_bits=16  bin_pt=0  align_bp=on  dbl_ovrd=off  block_type=logical
  Out1 : Outport
  wires:
  In1/1 -> Logical/1, Inverter1/1
  Logical/1 -> Out1/1
  Inverter1/1 -> Logical/2

== system exampleModel_bus_axi/example/dsp/Cav2/c1p1_PA_conversion/Subsystem3/posedge_pulse ==
  In1 : Inport
  Inverter1 : xbsIndex_r4/Inverter  en=off  latency=1  dbl_ovrd=off  block_type=inv
  Logical : xbsIndex_r4/Logical  logical_function=AND  inputs=2  en=off  latency=1  precision=Full  arith_type=Unsigned  n_bits=16  bin_pt=0  align_bp=on  dbl_ovrd=off  block_type=logical
  Out1 : Outport
  wires:
  Inverter1/1 -> Logical/2
  Logical/1 -> Out1/1
  In1/1 -> Inverter1/1, Logical/1

== system exampleModel_bus_axi/example/dsp/Cav2/c1p1_PA_conversion/Subsystem4/posedge_pulse ==
  In1 : Inport
  Inverter1 : xbsIndex_r4/Inverter  en=off  latency=1  dbl_ovrd=off  block_type=inv
  Logical : xbsIndex_r4/Logical  logical_function=AND  inputs=2  en=off  latency=1  precision=Full  arith_type=Unsigned  n_bits=16  bin_pt=0  align_bp=on  dbl_ovrd=off  block_type=logical
  Out1 : Outport
  wires:
  Inverter1/1 -> Logical/2
  Logical/1 -> Out1/1
  In1/1 -> Inverter1/1, Logical/1

== system exampleModel_bus_axi/example/dsp/Cav2/c1p1_PA_conversion1/Subsystem1/posedge_pulse ==
  In1 : Inport
  Inverter1 : xbsIndex_r4/Inverter  en=off  latency=1  dbl_ovrd=off  block_type=inv
  Logical : xbsIndex_r4/Logical  logical_function=AND  inputs=2  en=off  latency=1  precision=Full  arith_type=Unsigned  n_bits=16  bin_pt=0  align_bp=on  dbl_ovrd=off  block_type=logical
  Out1 : Outport
  wires:
  In1/1 -> Logical/1, Inverter1/1
  Logical/1 -> Out1/1
  Inverter1/1 -> Logical/2

== system exampleModel_bus_axi/example/dsp/Cav2/c1p1_PA_conversion1/Subsystem2/posedge_pulse ==
  In1 : Inport
  Inverter1 : xbsIndex_r4/Inverter  en=off  latency=1  dbl_ovrd=off  block_type=inv
  Logical : xbsIndex_r4/Logical  logical_function=AND  inputs=2  en=off  latency=1  precision=Full  arith_type=Unsigned  n_bits=16  bin_pt=0  align_bp=on  dbl_ovrd=off  block_type=logical
  Out1 : Outport
  wires:
  In1/1 -> Logical/1, Inverter1/1
  Logical/1 -> Out1/1
  Inverter1/1 -> Logical/2

== system exampleModel_bus_axi/example/dsp/Cav2/c1p1_PA_conversion1/Subsystem3/posedge_pulse ==
  In1 : Inport
  Inverter1 : xbsIndex_r4/Inverter  en=off  latency=1  dbl_ovrd=off  block_type=inv
  Logical : xbsIndex_r4/Logical  logical_function=AND  inputs=2  en=off  latency=1  precision=Full  arith_type=Unsigned  n_bits=16  bin_pt=0  align_bp=on  dbl_ovrd=off  block_type=logical
  Out1 : Outport
  wires:
  Inverter1/1 -> Logical/2
  Logical/1 -> Out1/1
  In1/1 -> Inverter1/1, Logical/1

== system exampleModel_bus_axi/example/dsp/Cav2/c1p1_PA_conversion1/Subsystem4/posedge_pulse ==
  In1 : Inport
  Inverter1 : xbsIndex_r4/Inverter  en=off  latency=1  dbl_ovrd=off  block_type=inv
  Logical : xbsIndex_r4/Logical  logical_function=AND  inputs=2  en=off  latency=1  precision=Full  arith_type=Unsigned  n_bits=16  bin_pt=0  align_bp=on  dbl_ovrd=off  block_type=logical
  Out1 : Outport
  wires:
  Inverter1/1 -> Logical/2
  Logical/1 -> Out1/1
  In1/1 -> Inverter1/1, Logical/1

== system exampleModel_bus_axi/example/dsp/Cav2/c1p2_freq_err_module1/freq_err1/delta_phi ==
  note: calculating delta phi
  phase : Inport
  window : Inport  Port=2
  reset : Inport  Port=3
  AddSub3 : xbsIndex_r4/AddSub  mode=Subtraction  use_carryin=off  use_carryout=off  en=on  latency=1  precision=Full  arith_type="Signed  (2's comp)"  n_bits=32  bin_pt=30  quantization=Truncate  overflow=Saturate  use_behavioral_HDL=off  hw_selection=Fabric  pipelined=off  dbl_ovrd=off  block_type=addsub
  Constant : xbsIndex_r4/Constant  const=0  gui_display_data_type=Fixed-point  arith_type=Signed (2's comp)  n_bits=1  bin_pt=0  preci_type=Single  exp_width=8  frac_width=24  explicit_period=off  period=1  equ=P=C  opselect=C  inp2=PCIN>>17  opr=+  inp1=P  carry=CIN  dbl_ovrd=off  block_type=constant
  Constant1 : xbsIndex_r4/Constant  const=0  gui_display_data_type=Fixed-point  arith_type=Signed (2's comp)  n_bits=1  bin_pt=0  preci_type=Single  exp_width=8  frac_width=24  explicit_period=off  period=1  equ=P=C  opselect=C  inp2=PCIN>>17  opr=+  inp1=P  carry=CIN  dbl_ovrd=off  block_type=constant
  Convert1 : xbsIndex_r4/Convert  gui_display_data_type=Boolean  arith_type=Boolean  n_bits=16  bin_pt=14  float_type=Single  exp_bits=8  fraction_bits=24  quantization=Truncate  overflow=Wrap  en=off  latency=1  pipeline=off  dbl_ovrd=off  block_type=convert
  Delay : xbsIndex_r4/Delay  rst=off  infoeditControl=Selection of Reset will increase slice count due to use of real FFs and instead of SRLs  en=off  latency=5  reg_retiming=off  dbl_ovrd=off  block_type=delay
  Delay2 : xbsIndex_r4/Delay  rst=off  infoeditControl=Selection of Reset will increase slice count due to use of real FFs and instead of SRLs  en=off  latency=2  reg_retiming=off  dbl_ovrd=off  block_type=delay
  Display : Display
  Display1 : Display
  Display2 : Display
  Gateway Out27 : xbsIndex_r4/Gateway Out  inherit_from_input=off  hdl_port=on  rows=1  columns=1  UseAsDAC=off  DACChannel='1'  interface=None  automatic_assignment=on  address_offset=hex2dec('00')  intf_name=''  intf_description=''  timing_constraint=None  locs_specified=off  LOCs={}  io_standard={}  block_type=gatewayout
  Gateway Out28 : xbsIndex_r4/Gateway Out  inherit_from_input=off  hdl_port=on  rows=1  columns=1  UseAsDAC=off  DACChannel='1'  interface=None  automatic_assignment=on  address_offset=hex2dec('00')  intf_name=''  intf_description=''  timing_constraint=None  locs_specified=off  LOCs={}  io_standard={}  block_type=gatewayout
  Gateway Out29 : xbsIndex_r4/Gateway Out  inherit_from_input=off  hdl_port=on  rows=1  columns=1  UseAsDAC=off  DACChannel='1'  interface=None  automatic_assignment=on  address_offset=hex2dec('00')  intf_name=''  intf_description=''  timing_constraint=None  locs_specified=off  LOCs={}  io_standard={}  block_type=gatewayout
  Inverter : xbsIndex_r4/Inverter  en=off  latency=1  dbl_ovrd=off  block_type=inv
  Logical : xbsIndex_r4/Logical  logical_function=AND  inputs=2  en=off  latency=7  precision=User Defined  arith_type=Boolean  n_bits=1  bin_pt=0  align_bp=on  dbl_ovrd=off  block_type=logical
  Relational : xbsIndex_r4/Relational  mode=a!=b  op_type=Bool  en=off  latency=1  dbl_ovrd=off  block_type=relational
  Relational1 : xbsIndex_r4/Relational  mode=a!=b  op_type=Bool  en=off  latency=1  dbl_ovrd=off  block_type=relational
  low_bit : Scope  NumInputPorts=4
  phase_latching : Subsystem
  posedge_pulse : Subsystem
  d_phi : Outport
  val_latched : Outport  Port=2
  wires:
  Delay/1 -> val_latched/1
  posedge_pulse/1(Out1) -> Delay/1
  reset/1 -> phase_latching/3(reset)
  Inverter/1 -> Delay2/1
  Delay2/1 -> AddSub3/3
  Gateway Out29/1 -> low_bit/1, Display/1
  phase/1 -> phase_latching/1(phase)
  AddSub3/1 -> Gateway Out27/1, d_phi/1
  Gateway Out28/1 -> low_bit/2, Display1/1
  Gateway Out27/1 -> low_bit/3, Display2/1
  Convert1/1 -> Inverter/1
  window/1 -> Convert1/1, phase_latching/2(window)
  phase_latching/1(Stop_value) -> AddSub3/1, Relational/1, Gateway Out29/1
  Constant/1 -> Relational/2
  Constant1/1 -> Relational1/2
  phase_latching/2(Start_value) -> Relational1/1, Gateway Out28/1, AddSub3/2
  Relational/1 -> Logical/1
  Relational1/1 -> Logical/2
  Logical/1 -> posedge_pulse/1(In1)

== system exampleModel_bus_axi/example/dsp/Cav2/c1p2_freq_err_module1/freq_err1/delta_t ==
  note: (2*pi)/(17E6)
  window : Inport
  reset : Inport  Port=2
  Constant1 : xbsIndex_r4/Constant  const=2*pi*(1/(Fsig))  gui_display_data_type=Fixed-point  arith_type=Unsigned  n_bits=42  bin_pt=42  preci_type=Single  exp_width=8  frac_width=24  explicit_period=off  period=1  equ=P=C  opselect=C  inp2=PCIN>>17  opr=+  inp1=P  carry=CIN  dbl_ovrd=off  block_type=constant
  Convert1 : xbsIndex_r4/Convert  gui_display_data_type=Boolean  arith_type=Boolean  n_bits=16  bin_pt=14  float_type=Single  exp_bits=8  fraction_bits=24  quantization=Truncate  overflow=Wrap  en=off  latency=1  pipeline=off  dbl_ovrd=off  block_type=convert
  Counter2 : xbsIndex_r4/Counter  cnt_type=Free Running  cnt_to=Inf  operation=Up  start_count=1  cnt_by_val=1  arith_type=Unsigned  n_bits=10  bin_pt=0  load_pin=off  rst=on  en=on  explicit_period=on  period=1/(17e6)  use_behavioral_HDL=off  implementation=Fabric  dbl_ovrd=off  block_type=counter
  Delay : xbsIndex_r4/Delay  rst=off  infoeditControl=Selection of Reset will increase slice count due to use of real FFs and instead of SRLs  en=off  latency=1  reg_retiming=off  dbl_ovrd=off  block_type=delay
  Display1 : Display
  Display3 : Display
  Gateway Out1 : xbsIndex_r4/Gateway Out  inherit_from_input=off  hdl_port=on  rows=1  columns=1  UseAsDAC=off  DACChannel='1'  interface=None  automatic_assignment=on  address_offset=hex2dec('00')  intf_name=''  intf_description=''  timing_constraint=None  locs_specified=off  LOCs={}  io_standard={}  block_type=gatewayout
  Gateway Out6 : xbsIndex_r4/Gateway Out  inherit_from_input=off  hdl_port=on  rows=1  columns=1  UseAsDAC=off  DACChannel='1'  interface=None  automatic_assignment=on  address_offset=hex2dec('00')  intf_name=''  intf_description=''  timing_constraint=None  locs_specified=off  LOCs={}  io_standard={}  block_type=gatewayout
  Mult1 : xbsIndex_r4/Mult  precision=User Defined  arith_type="Signed  (2's comp)"  n_bits=32  bin_pt=32  quantization=Truncate  overflow=Saturate  en=off  latency=3  use_behavioral_HDL=off  opt=Speed  use_embedded=on  optimum_pipeline=off  pipeline=on  dbl_ovrd=off  use_rpm=on  placement_style=Triangular  block_type=mult
  Register2 : xbsIndex_r4/Register  init=0  rst=on  en=on  dbl_ovrd=off  block_type=register
  dt : Outport
  wires:
  Constant1/1 -> Mult1/2
  Mult1/1 -> dt/1, Gateway Out1/1
  reset/1 -> Register2/2, Counter2/1
  Register2/1 -> Gateway Out6/1, Mult1/1
  Counter2/1 -> Register2/1
  window/1 -> Convert1/1
  Gateway Out1/1 -> Display3/1
  Gateway Out6/1 -> Display1/1
  Convert1/1 -> Delay/1
  Delay/1 -> Register2/3, Counter2/2

== system exampleModel_bus_axi/example/dsp/Cav2/c1p2_freq_err_module1/freq_err1/negedge_pulse ==
  In1 : Inport
  Delay3 : xbsIndex_r4/Delay  rst=off  infoeditControl=Selection of Reset will increase slice count due to use of real FFs and instead of SRLs  en=off  latency=4  reg_retiming=off  dbl_ovrd=off  block_type=delay
  Inverter : xbsIndex_r4/Inverter  en=off  latency=1  dbl_ovrd=off  block_type=inv
  Logical : xbsIndex_r4/Logical  logical_function=AND  inputs=2  en=off  latency=1  precision=Full  arith_type=Unsigned  n_bits=16  bin_pt=0  align_bp=on  dbl_ovrd=off  block_type=logical
  Out1 : Outport
  wires:
  Delay3/1 -> Logical/2
  Logical/1 -> Out1/1
  Inverter/1 -> Logical/1
  In1/1 -> Delay3/1, Inverter/1

== system exampleModel_bus_axi/example/dsp/Cav2/c1p2_freq_err_module1/freq_err1/posedge_pulse ==
  In1 : Inport
  Inverter1 : xbsIndex_r4/Inverter  en=off  latency=1  dbl_ovrd=off  block_type=inv
  Logical : xbsIndex_r4/Logical  logical_function=AND  inputs=2  en=off  latency=1  precision=Full  arith_type=Unsigned  n_bits=16  bin_pt=0  align_bp=on  dbl_ovrd=off  block_type=logical
  Out1 : Outport
  wires:
  In1/1 -> Logical/1, Inverter1/1
  Logical/1 -> Out1/1
  Inverter1/1 -> Logical/2
